simulink model "HW1_Simulink"  (R2021a)
settings: Solver=FixedStepAuto  StartTime=0.0  StopTime=50.0  FixedStep=0.002  RelTol=1e-3
settings Model: Creator=Personal Account  LastModifiedBy=Personal Account

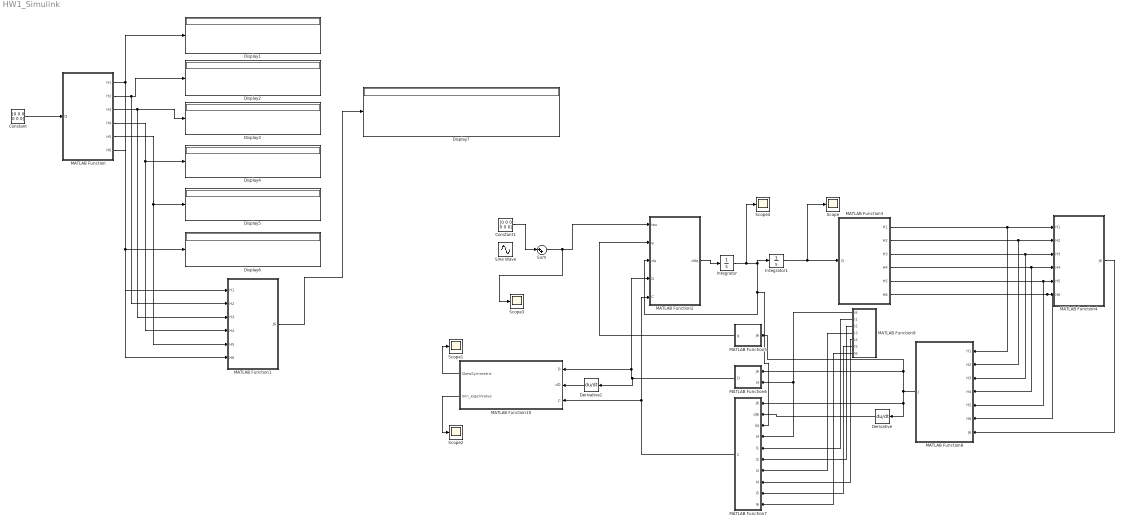
== system HW1_Simulink ==
  Constant : Constant  Value=[0 0 0 0 0 0]
  Constant1 : Constant  Value=[0 0 0 0 0 0]
  Derivative : Derivative  CoefficientInTFapproximation=0.001
  Derivative1 : Derivative  CoefficientInTFapproximation=0.001
  Display{1..7} (7 alike) : Display
  Integrator : Integrator  InitialCondition=[0;0;0;0;0;0]
  Integrator1 : Integrator  InitialCondition=[0;pi/2;0;0;0;0]
  MATLAB Function : MATLAB Function  TreatAsAtomicUnit=on
  MATLAB Function1 : MATLAB Function  TreatAsAtomicUnit=on
  MATLAB Function10 : MATLAB Function  TreatAsAtomicUnit=on
  MATLAB Function2 : MATLAB Function  TreatAsAtomicUnit=on
  MATLAB Function3 : MATLAB Function  TreatAsAtomicUnit=on
  MATLAB Function4 : MATLAB Function  TreatAsAtomicUnit=on
  MATLAB Function5 : MATLAB Function  TreatAsAtomicUnit=on
  MATLAB Function6 : MATLAB Function  TreatAsAtomicUnit=on
  MATLAB Function7 : MATLAB Function  TreatAsAtomicUnit=on
  MATLAB Function8 : MATLAB Function  TreatAsAtomicUnit=on
  MATLAB Function9 : MATLAB Function  TreatAsAtomicUnit=on
  Scope{,1..4} (5 alike) : Scope
  Sine Wave : Sin  Amplitude=[1;0;0;0;0;0]  SampleTime=0  VectorParams1D=off
  Sum : Sum  Inputs=|++
  wires:
  Constant/1 -> MATLAB Function/1(Q)
  MATLAB Function/1(H1) -> Display1/1, MATLAB Function1/1(H1)
  MATLAB Function/6(H6) -> MATLAB Function1/6(H6), Display6/1
  MATLAB Function/5(H5) -> MATLAB Function1/5(H5), Display5/1
  MATLAB Function/4(H4) -> Display4/1, MATLAB Function1/4(H4)
  MATLAB Function/3(H3) -> MATLAB Function1/3(H3), Display3/1
  MATLAB Function/2(H2) -> Display2/1, MATLAB Function1/2(H2)
  MATLAB Function1/1(J6) -> Display7/1
  MATLAB Function2/1(ddq) -> Integrator/1
  Integrator1/1 -> Scope/1, MATLAB Function3/1(Q)
  MATLAB Function3/6(H6) -> MATLAB Function8/6(H6), MATLAB Function4/6(H6)
  MATLAB Function3/5(H5) -> MATLAB Function8/5(H5), MATLAB Function4/5(H5)
  MATLAB Function3/4(H4) -> MATLAB Function8/4(H4), MATLAB Function4/4(H4)
  MATLAB Function3/3(H3) -> MATLAB Function8/3(H3), MATLAB Function4/3(H3)
  MATLAB Function3/2(H2) -> MATLAB Function8/2(H2), MATLAB Function4/2(H2)
  MATLAB Function3/1(H1) -> MATLAB Function8/1(H1), MATLAB Function4/1(H1)
  Integrator/1 -> Scope4/1, Integrator1/1, MATLAB Function2/3(dq), MATLAB Function7/3(dq)
  Derivative/1 -> MATLAB Function7/2(dJ6)
  MATLAB Function7/1(C) -> MATLAB Function10/3(C), MATLAB Function2/5(C)
  MATLAB Function6/1(D) -> Derivative1/1, MATLAB Function10/1(D), MATLAB Function2/4(D)
  MATLAB Function5/1(g) -> MATLAB Function2/2(g)
  MATLAB Function8/1(J) -> Derivative/1, MATLAB Function7/1(J6), MATLAB Function6/1(J6), MATLAB Function5/1(J6)
  MATLAB Function4/1(J6) -> MATLAB Function8/7(J6)
  MATLAB Function9/1(M) -> MATLAB Function7/4(M), MATLAB Function6/2(M)
  MATLAB Function9/2(I1) -> MATLAB Function7/5(I1)
  MATLAB Function9/3(I2) -> MATLAB Function7/6(I2)
  MATLAB Function9/4(I3) -> MATLAB Function7/7(I3)
  MATLAB Function9/5(I4) -> MATLAB Function7/8(I4)
  MATLAB Function9/6(I5) -> MATLAB Function7/9(I5)
  MATLAB Function9/7(I6) -> MATLAB Function7/10(I6)
  Derivative1/1 -> MATLAB Function10/2(dD)
  MATLAB Function10/1(SkewSymmetric) -> Scope1/1
  MATLAB Function10/2(min_eigenValue) -> Scope2/1
  Sum/1 -> Scope3/1, MATLAB Function2/1(tau)
  Constant1/1 -> Sum/1

== matlab function HW1_Simulink/MATLAB Function7 ==
  data: J6 input; dJ6 input; C output; dq input; M input; I1 input; I2 input; I3 input; I4 input; I5 input; I6 input
function C  = C(J6,dJ6,dq, M, I1, I2, I3, I4, I5, I6)    
    w = J6*dq;
    w = w(19:36);
    S = zeros(36);
    S(19:21,19:21) = -skew(I1*w(1:3));
    S(22:24,22:24) = -skew(I2*w(4:6));
    S(25:27,25:27) = -skew(I3*w(7:9));
    S(28:30,28:30) = -skew(I4*w(10:12));
    S(31:33,31:33) = -skew(I5*w(13:15));
    S(34:36,34:36) = -skew(I6*w(16:18));
    
    C = transpose(J6) * M * dJ6 + transpose(J6) * S * J6;

== matlab function HW1_Simulink/MATLAB Function8 ==
  data: H1 input; H2 input; H3 input; H4 input; H5 input; H6 input; J6 input; J output
function J  = generalized_J(H1, H2, H3, H4, H5, H6, J6)
    Jv = J6(1:3,1:6);
    Jw = J6(4:6,1:6);
    
    x=[1;0;0];
    y=[0;1;0];
    z=[0;0;1];
    
    rcd_1 = H1(1:3,1:3) * 0.396/2 *(-y);
    rcd_2 = H2(1:3,1:3) * 0.324/2 * x;
    rcd_3 = H3(1:3,1:3) * 0.343/6 * z;
    rcd_4 = H4(1:3,1:3) * 0.343/4 * y;
    rcd_5 = H5(1:3,1:3) * 0.165/2 * z;
    rcd_6 = [0;0;0];
    
    J = [skew(rcd_1) * [Jw(:,1) zeros(3,5)] + [Jv(:,1) zeros(3,5)];
         skew(rcd_2) * [Jw(:,1:2) zeros(3,4)] + [Jv(:,1:2) zeros(3,4)];
         skew(rcd_3) * [Jw(:,1:3) zeros(3,3)] + [Jv(:,1:3) zeros(3,3)];
         skew(rcd_4) * [Jw(:,1:4) zeros(3,2)] + [Jv(:,1:4) zeros(3,2)];
         skew(rcd_5) * [Jw(:,1:5) zeros(3,1)] + [Jv(:,1:5) zeros(3,1)];
         skew(rcd_6) * Jw(:,1:6) + Jv(:,1:6);
         (H1(1:3,1:3)^(-1))*[Jw(:,1) zeros(3,5)];
         (H2(1:3,1:3)^(-1))*[Jw(:,1:2) zeros(3,4)];
         (H3(1:3,1:3)^(-1))*[Jw(:,1:3) zeros(3,3)];
         (H4(1:3,1:3)^(-1))*[Jw(:,1:4) zeros(3,2)];
         (H5(1:3,1:3)^(-1))*[Jw(:,1:5) zeros(3,1)];
         (H6(1:3,1:3)^(-1))*Jw(:,1:6)];

== matlab function HW1_Simulink/MATLAB Function9 ==
  data: M output; I1 output; I2 output; I3 output; I4 output; I5 output; I6 output
function [M, I1, I2, I3, I4, I5, I6]  = M()
    M = zeros(36);
    M(1:3,1:3) = eye(3) * 10;
    M(4:6,4:6) = eye(3) * 10;
    M(7:9,7:9) = eye(3) * 10;
    M(10:12,10:12) = eye(3) * 5;
    M(13:15,13:15) = eye(3) * 5;
    M(16:18,16:18) = eye(3) * 5;
    r = 172/4/1000;
%     M(21,21) = 0.5*10*r^2;
%     M(24,24) = 0.5*10*r^2;
%     M(27,27) = 0.5*10*r^2;
%     M(30,30) = 0.5*5*r^2;
%     M(33,33) = 0.5*5*r^2;
%     M(36,36) = 0.5*5*r^2;
    m1=10/2; m2=5/2;
    I1 = [0 0 0;0 0 0;0 0 2*m1*(0.396/2)^2 + 2*1/2*m1*r^2];
    I2 = [0 0 0;0 0 0;2 0 2*m1*(0.324/2)^2 + 2*1/2*m1*r^2];
    I3 = [0 0 0;0 0 0;0 0 m1*(0.343/2*1/3)^2+m2*(0.343/2*2/3)^2 + 1/2*m1*r^2 + 1/2*m2*r^2];
    I4 = [0 0 0;0 0 0;0 0 2*m2*(0.343/4)^2 + 2*1/2*m2*r^2];
    I5 = [0 0 0;0 0 0;0 0 2*m2*(0.165/2)^2 + 2*1/2*m2*r^2];
    I6 = [0 0 0;0 0 0;0 0 1/2*m2*r^2];
    M(19:21,19:21) = I1;
    M(22:24,22:24) = I2;
    M(25:27,25:27) = I3;
    M(28:30,28:30) = I4;
    M(31:33,31:33) = I5;
    M(34:36,34:36) = I6;

== matlab function HW1_Simulink/MATLAB Function10 ==
  data: D input; SkewSymmetric output; dD input; C input; min_eigenValue output
function [SkewSymmetric, min_eigenValue]  = Positive_Definit(D,dD,C)    
    SkewSymmetric = [1 2 3 4 5 6] * (dD-2*C) * [1;2;3;4;5;6];
    EigenV = eig(D);
    min_eigenValue = min(EigenV);

== matlab function HW1_Simulink/MATLAB Function1 ==
  data: H1 input; J6 output; H2 input; H3 input; H4 input; H5 input; H6 input
function J6  = J(H1, H2, H3, H4, H5, H6)
    k = [0;0;1];
    jw = [k H1(1:3,1:3)*k H2(1:3,1:3)*k H3(1:3,1:3)*k H4(1:3,1:3)*k H5(1:3,1:3)*k];
    jv = [cross(k,H6(1:3,4)-[0;0;0]) cross(H1(1:3,1:3)*k,H6(1:3,4)-H1(1:3,4)) cross(H2(1:3,1:3)*k,H6(1:3,4)-H2(1:3,4)) ...
          cross(H3(1:3,1:3)*k,H6(1:3,4)-H3(1:3,4)) cross(H4(1:3,1:3)*k,H6(1:3,4)-H4(1:3,4)) cross(H5(1:3,1:3)*k,H6(1:3,4)-H5(1:3,4))];
    J6 = [jv;jw];

== matlab function HW1_Simulink/MATLAB Function ==
  data: Q input; H1 output; H2 output; H3 output; H4 output; H5 output; H6 output
function [H1, H2, H3, H4, H5, H6] = H(Q)
    T1 = [cos(Q(1)) -sin(Q(1)) 0 0;
          sin(Q(1)) cos(Q(1))  0 0;
          0         0          1 0;
          0         0          0 1];
      
    T2 = [1         0          0 0;
          0         1          0 0;
          0         0          1 0.396;
          0         0          0 1];
      
    T3 = [1         0          0 00;
          0         1          0 0;
          0         0          1 0;
          0         0          0 1];
      
    T4 = [1         0            0 0;
          0         cos(-pi/2)   -sin(-pi/2) 0;
          0         sin(-pi/2)   cos(-pi/2)  0;
          0         0            0           1];
    H1 = T1 * T2 * T3 * T4;
    
    T1 = [cos(Q(2)) -sin(Q(2)) 0 0;
          sin(Q(2)) cos(Q(2))  0 0;
          0         0          1 0;
          0         0          0 1];
      
    T2 = [1         0          0 0;
          0         1          0 0;
          0         0          1 0;
          0         0          0 1];
      
    T3 = [1         0          0 0.324;
          0         1          0 0;
          0         0          1 0;
          0         0          0 1];
      
    T4 = [1         0            0 0;
          0         cos(0)   -sin(0) 0;
          0         sin(0)   cos(0)  0;
          0         0            0           1];
    H2 = H1 * T1 * T2 * T3 * T4;
    
    T1 = [cos(Q(3)) -sin(Q(3)) 0 0;
          sin(Q(3)) cos(Q(3))  0 0;
          0         0          1 0;
          0         0          0 1];
      
    T2 = [1         0          0 0;
          0         1          0 0;
          0         0          1 0;
          0         0          0 1];
      
    T3 = [1         0          0 0;
          0         1          0 0;
          0         0          1 0;
          0         0          0 1];
      
    T4 = [1         0            0 0;
          0         cos(-pi/2)   -sin(-pi/2) 0;
          0         sin(-pi/2)   cos(-pi/2)  0;
          0         0            0           1];
    H3 = H2 * T1 * T2 * T3 * T4;
    
    T1 = [cos(Q(4)) -sin(Q(4)) 0 0;
          sin(Q(4)) cos(Q(4))  0 0;
          0         0          1 0;
          0         0          0 1];
      
    T2 = [1         0          0 0;
          0         1          0 0;
          0         0          1 0.343;
          0         0          0 1];
      
    T3 = [1         0          0 0;
          0         1          0 0;
          0         0          1 0;
          0         0          0 1];
      
    T4 = [1         0            0 0;
          0         cos(pi/2)   -sin(pi/2) 0;
          0         sin(pi/2)   cos(pi/2)  0;
          0         0            0           1];
    H4 = H3 * T1 * T2 * T3 * T4;
    
    T1 = [cos(Q(5)) -sin(Q(5)) 0 0;
          sin(Q(5)) cos(Q(5))  0 0;
          0         0          1 0;
          0         0          0 1];
      
    T2 = [1         0          0 0;
          0         1          0 0;
          0         0          1 0;
          0         0          0 1];
      
    T3 = [1         0          0 0;
          0         1          0 0;
          0         0          1 0;
          0         0          0 1];
      
    T4 = [1         0            0 0;
          0         cos(pi/2)   -sin(pi/2) 0;
          0         sin(pi/2)   cos(pi/2)  0;
          0         0            0           1];
    H5 = H4 * T1 * T2 * T3 * T4;
    
    T1 = [cos(Q(6)) -sin(Q(6)) 0 0;
          sin(Q(6)) cos(Q(6))  0 0;
          0         0          1 0;
          0         0          0 1];
      
    T2 = [1         0          0 0;
          0         1          0 0;
          0         0          1 0.165;
          0         0          0 1];
      
    T3 = [1         0          0 0;
          0         1          0 0;
          0         0          1 0;
          0         0          0 1];
      
    T4 = [1         0            0 0;
          0         cos(0)   -sin(0) 0;
          0         sin(0)   cos(0)  0;
          0         0            0           1];
    H6 = H5 * T1 * T2 * T3 * T4;

== matlab function HW1_Simulink/MATLAB Function2 ==
  data: tau input; g input; dq input; ddq output; D input; C input
function ddq  = Robot_model(tau,g,dq,D,C)
    ddq = D^(-1) * (tau - C * dq - g);

== matlab function HW1_Simulink/MATLAB Function3 ==
  data: Q input; H1 output; H2 output; H3 output; H4 output; H5 output; H6 output
function [H1, H2, H3, H4, H5, H6] = H(Q)
    T1 = [cos(Q(1)) -sin(Q(1)) 0 0;
          sin(Q(1)) cos(Q(1))  0 0;
          0         0          1 0;
          0         0          0 1];
      
    T2 = [1         0          0 0;
          0         1          0 0;
          0         0          1 0.396;
          0         0          0 1];
      
    T3 = [1         0          0 00;
          0         1          0 0;
          0         0          1 0;
          0         0          0 1];
      
    T4 = [1         0            0 0;
          0         cos(-pi/2)   -sin(-pi/2) 0;
          0         sin(-pi/2)   cos(-pi/2)  0;
          0         0            0           1];
    H1 = T1 * T2 * T3 * T4;
    
    T1 = [cos(Q(2)) -sin(Q(2)) 0 0;
          sin(Q(2)) cos(Q(2))  0 0;
          0         0          1 0;
          0         0          0 1];
      
    T2 = [1         0          0 0;
          0         1          0 0;
          0         0          1 0;
          0         0          0 1];
      
    T3 = [1         0          0 0.324;
          0         1          0 0;
          0         0          1 0;
          0         0          0 1];
      
    T4 = [1         0            0 0;
          0         cos(0)   -sin(0) 0;
          0         sin(0)   cos(0)  0;
          0         0            0           1];
    H2 = H1 * T1 * T2 * T3 * T4;
    
    T1 = [cos(Q(3)) -sin(Q(3)) 0 0;
          sin(Q(3)) cos(Q(3))  0 0;
          0         0          1 0;
          0         0          0 1];
      
    T2 = [1         0          0 0;
          0         1          0 0;
          0         0          1 0;
          0         0          0 1];
      
    T3 = [1         0          0 0;
          0         1          0 0;
          0         0          1 0;
          0         0          0 1];
      
    T4 = [1         0            0 0;
          0         cos(-pi/2)   -sin(-pi/2) 0;
          0         sin(-pi/2)   cos(-pi/2)  0;
          0         0            0           1];
    H3 = H2 * T1 * T2 * T3 * T4;
    
    T1 = [cos(Q(4)) -sin(Q(4)) 0 0;
          sin(Q(4)) cos(Q(4))  0 0;
          0         0          1 0;
          0         0          0 1];
      
    T2 = [1         0          0 0;
          0         1          0 0;
          0         0          1 0.343;
          0         0          0 1];
      
    T3 = [1         0          0 0;
          0         1          0 0;
          0         0          1 0;
          0         0          0 1];
      
    T4 = [1         0            0 0;
          0         cos(pi/2)   -sin(pi/2) 0;
          0         sin(pi/2)   cos(pi/2)  0;
          0         0            0           1];
    H4 = H3 * T1 * T2 * T3 * T4;
    
    T1 = [cos(Q(5)) -sin(Q(5)) 0 0;
          sin(Q(5)) cos(Q(5))  0 0;
          0         0          1 0;
          0         0          0 1];
      
    T2 = [1         0          0 0;
          0         1          0 0;
          0         0          1 0;
          0         0          0 1];
      
    T3 = [1         0          0 0;
          0         1          0 0;
          0         0          1 0;
          0         0          0 1];
      
    T4 = [1         0            0 0;
          0         cos(pi/2)   -sin(pi/2) 0;
          0         sin(pi/2)   cos(pi/2)  0;
          0         0            0           1];
    H5 = H4 * T1 * T2 * T3 * T4;
    
    T1 = [cos(Q(6)) -sin(Q(6)) 0 0;
          sin(Q(6)) cos(Q(6))  0 0;
          0         0          1 0;
          0         0          0 1];
      
    T2 = [1         0          0 0;
          0         1          0 0;
          0         0          1 0.165;
          0         0          0 1];
      
    T3 = [1         0          0 0;
          0         1          0 0;
          0         0          1 0;
          0         0          0 1];
      
    T4 = [1         0            0 0;
          0         cos(0)   -sin(0) 0;
          0         sin(0)   cos(0)  0;
          0         0            0           1];
    H6 = H5 * T1 * T2 * T3 * T4;

== matlab function HW1_Simulink/MATLAB Function4 ==
  data: H1 input; J6 output; H2 input; H3 input; H4 input; H5 input; H6 input
function J6  = J(H1, H2, H3, H4, H5, H6)
    k = [0;0;1];
    jw = [k H1(1:3,1:3)*k H2(1:3,1:3)*k H3(1:3,1:3)*k H4(1:3,1:3)*k H5(1:3,1:3)*k];
    jv = [cross(k,H6(1:3,4)-[0;0;0]) cross(H1(1:3,1:3)*k,H6(1:3,4)-H1(1:3,4)) cross(H2(1:3,1:3)*k,H6(1:3,4)-H2(1:3,4)) ...
          cross(H3(1:3,1:3)*k,H6(1:3,4)-H3(1:3,4)) cross(H4(1:3,1:3)*k,H6(1:3,4)-H4(1:3,4)) cross(H5(1:3,1:3)*k,H6(1:3,4)-H5(1:3,4))];
    J6 = [jv;jw];

== matlab function HW1_Simulink/MATLAB Function5 ==
  data: J6 input; g output
function g  = g(J6)
    g0 = zeros(36,1);
    g0(3) = 9.8 * 10;
    g0(6) = 9.8 * 10;
    g0(9) = 9.8 * 10;
    g0(12) = 9.8 * 5;
    g0(15) = 9.8 * 5;
    g0(18) = 9.8 * 5;
    g = transpose(J6) * g0;

== matlab function HW1_Simulink/MATLAB Function6 ==
  data: J6 input; D output; M input
function D  = D(J6,M)    
    D = transpose(J6) * M * J6;
